simulink model "Linear_Model_Check_mks_4Nov_maininput_cruise"  (R2022b)
settings: Solver=VariableStepAuto  StartTime=0.0  StopTime=3240  FixedStep=0.5  RelTol=1e-6
settings Model: Creator=Mitarbeiter  LastModifiedBy=Mitarbeiter

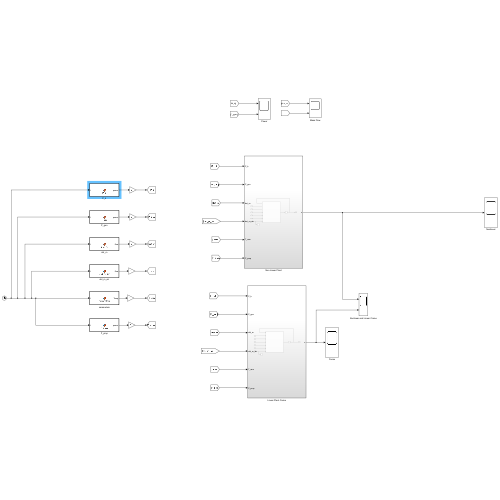
[thumbnail: Simulink's stored preview of the top-level diagram]
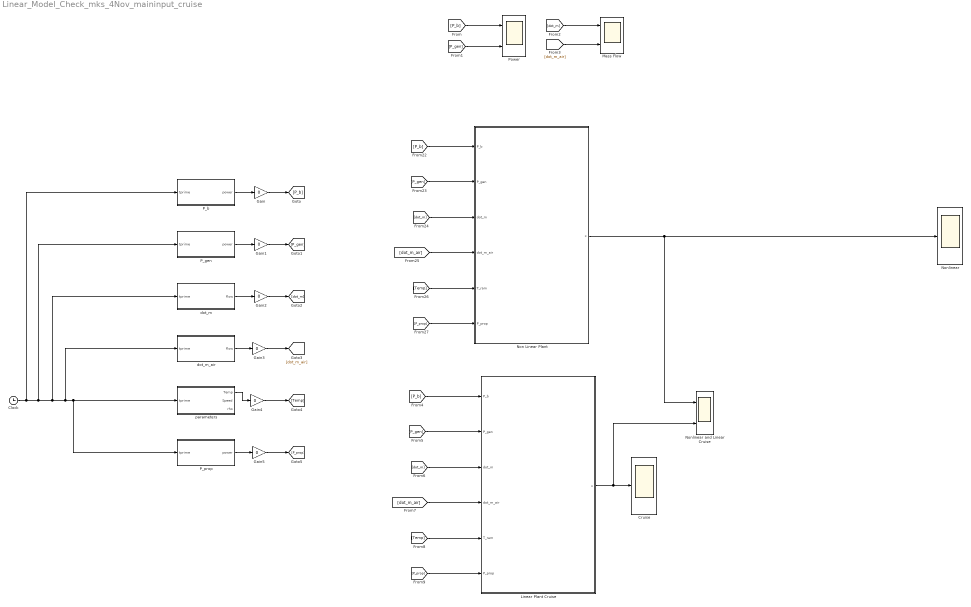
== system Linear_Model_Check_mks_4Nov_maininput_cruise ==
  Clock : Clock
  Cruise : Scope
  Gain{,1..5} (6 alike) : Gain  Gain=0
  Linear Plant Cruise : Subsystem
  Mass Flow : Scope  NumInputPorts=2
  Non Linear Plant : Subsystem
  Nonlinear : Scope
  Nonlinear and Linear Cruise : Scope  NumInputPorts=2
  P_b : MATLAB Function  TreatAsAtomicUnit=on
  P_gen : MATLAB Function  TreatAsAtomicUnit=on
  P_prop : MATLAB Function  TreatAsAtomicUnit=on
  Power : Scope  NumInputPorts=2
  dot_m : MATLAB Function  TreatAsAtomicUnit=on
  dot_m_air : MATLAB Function  TreatAsAtomicUnit=on
  parameters : MATLAB Function  TreatAsAtomicUnit=on
  wires:
  [P_b] -> Power/1
  [P_gen] -> Power/2
  [dot_m] -> Mass Flow/1
  [dot_m_air] -> Mass Flow/2
  [P_b] -> Linear Plant Cruise/1(P_b)
  [dot_m] -> Linear Plant Cruise/3(dot_m)
  Linear Plant Cruise/1(x) -> Nonlinear and Linear Cruise/2, Cruise/1
  [Temp] -> Linear Plant Cruise/5(T_ram)
  [P_prop] -> Linear Plant Cruise/6(P_prop)
  [dot_m_air] -> Linear Plant Cruise/4(dot_m_air)
  [P_gen] -> Linear Plant Cruise/2(P_gen)
  Gain5/1 -> [P_prop]
  P_b/1(power) -> Gain/1
  Gain2/1 -> [dot_m]
  Gain/1 -> [P_b]
  Gain1/1 -> [P_gen]
  P_gen/1(power) -> Gain1/1
  Gain3/1 -> [dot_m_air]
  P_prop/1(power) -> Gain5/1
  parameters/1(Temp) -> Gain4/1
  Clock/1 -> P_b/1(tprime), P_gen/1(tprime), dot_m/1(tprime), dot_m_air/1(tprime), parameters/1(tprime), P_prop/1(tprime)
  Gain4/1 -> [Temp]
  dot_m/1(flow) -> Gain2/1
  dot_m_air/1(flow) -> Gain3/1
  [P_b] -> Non Linear Plant/1(P_b)
  [dot_m] -> Non Linear Plant/3(dot_m)
  Non Linear Plant/1(x) -> Nonlinear and Linear Cruise/1, Nonlinear/1
  [Temp] -> Non Linear Plant/5(T_ram)
  [P_prop] -> Non Linear Plant/6(P_prop)
  [dot_m_air] -> Non Linear Plant/4(dot_m_air)
  [P_gen] -> Non Linear Plant/2(P_gen)

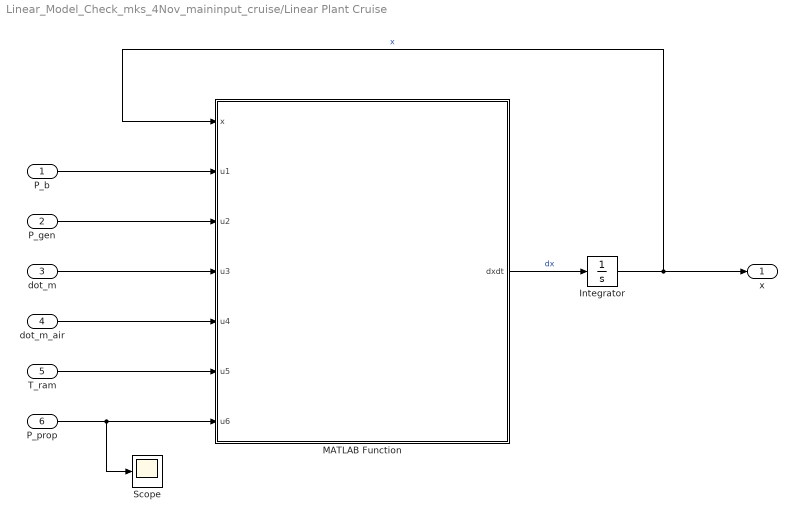
== system Linear_Model_Check_mks_4Nov_maininput_cruise/Linear Plant Cruise ==
  P_b : Inport
  P_gen : Inport  Port=2
  dot_m : Inport  Port=3
  dot_m_air : Inport  Port=4
  T_ram : Inport  Port=5
  P_prop : Inport  Port=6
  Integrator : Integrator  InitialCondition=[52814776030872794621339/2111078349043945281000; 104094200346052350023/4282106184673317000; 0.95; 7429519190417529794477/301582621291992183000; 14970426814841764289/611729454953331000; 62413813461003262061339/2111078349043945281000; 115709353125739950023/4282106184673317000; 1317031521595249/55809639171000; 192210910256741628225757/6125247032447703303000; 18157083865504564289/611729454953331000; 1317031521595249/55809639171000; 29037669531913/1240214203800; 1405698391771/60204573000];
  MATLAB Function : MATLAB Function  TreatAsAtomicUnit=on
  Scope : Scope
  x : Outport
  wires:
  MATLAB Function/1(dxdt) -> Integrator/1  "dx"
  Integrator/1 -> x/1, MATLAB Function/1(x)  "x"
  P_prop/1 -> Scope/1, MATLAB Function/7(u6)
  P_b/1 -> MATLAB Function/2(u1)
  P_gen/1 -> MATLAB Function/3(u2)
  dot_m/1 -> MATLAB Function/4(u3)
  dot_m_air/1 -> MATLAB Function/5(u4)
  T_ram/1 -> MATLAB Function/6(u5)

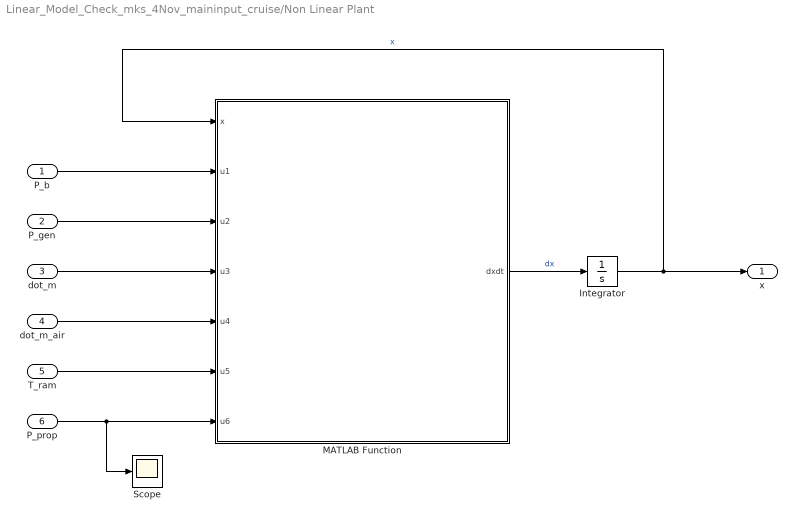
== system Linear_Model_Check_mks_4Nov_maininput_cruise/Non Linear Plant ==
  P_b : Inport
  P_gen : Inport  Port=2
  dot_m : Inport  Port=3
  dot_m_air : Inport  Port=4
  T_ram : Inport  Port=5
  P_prop : Inport  Port=6
  Integrator : Integrator  InitialCondition=[93988057444394599308387229/4422589792359066198000000; 14175896344014406900981/690059259222822000000; 0.95; 642296550198010131218710603/30958128546513463386000000; 99794188918686328306867/4830414814559754000000; 20; 748871653711516104483208603/30958128546513463386000000; 109523475430206270118867/4830414814559754000000; 20; 114489338227757388521/5840888530302000000; 20; 1232797079008717771442215271/48366943538186816802000000; 118698981952749594118867/4830414814559754000000; 114489338227757388521/5840888530302000000; 1053909433374709813/54082301206500000; 8752431102689/450060759000]
  MATLAB Function : MATLAB Function  TreatAsAtomicUnit=on
  Scope : Scope
  x : Outport
  wires:
  MATLAB Function/1(dxdt) -> Integrator/1  "dx"
  Integrator/1 -> x/1, MATLAB Function/1(x)  "x"
  P_prop/1 -> Scope/1, MATLAB Function/7(u6)
  P_b/1 -> MATLAB Function/2(u1)
  P_gen/1 -> MATLAB Function/3(u2)
  dot_m/1 -> MATLAB Function/4(u3)
  dot_m_air/1 -> MATLAB Function/5(u4)
  T_ram/1 -> MATLAB Function/6(u5)

== matlab function Linear_Model_Check_mks_4Nov_maininput_cruise/Linear Plant Cruise/MATLAB Function ==
  data: x input; dxdt output; u1 input; u2 input; u3 input; u4 input; u5 input; u6 input
function dxdt = fcn(x,u1,u2,u3,u4,u5,u6)

u = [u1;u2;u3;u4;u5;u6];
dxdt = aircraft_dynamics_linear_cruise(x,u);

== matlab function Linear_Model_Check_mks_4Nov_maininput_cruise/P_b ==
  data: tprime input; power output
function power = P_b_0to3240(tprime)
% Rebase original profile window: new t' in [0, 3240] corresponds to original t = t' + 421

    % --- Power values (same as your original code) ---
    power_values = [541728.972461324, 525434.547259656, 484698.484257782, ...
                    443962.421182278, 403226.358083855, 362490.295190934, ...
                    321754.232292711, 281018.169380235, 240282.106417171, ...
                    199546.043463649, 158809.980492022, 118073.917524794, ...
                    77337.8545513178, 36601.7915815174, 4012.94120061964, ...
                    4012.94120060897, 4012.94120058611, 4012.94120055903, ...
                    4012.94120053569, 4012.94120052215, 4012.94120051169, ...
                    4012.94120050506, 4012.94120050103, 4012.94120049878, ...
                    4012.94120049977, 4012.94120050145, 4012.94120050538, ...
                    4012.94120051198, 4012.94120052045, 4012.94120053546, ...
                    4012.94120055757, 4012.94120058035, 4012.94120057094, ...
                    9.73312208790910e-10, -3.25790856001986e-10, ...
                    -7.33764827360896e-10, -3.22870604452897e-11, ...
                    -2.89901400312855e-11, -6.19593223381754e-11, ...
                    -4.77143652162351e-10, 3.07295526727322e-10, ...
                    -5.97594860992170e-10, 7.70455739254353e-10, ...
                    -4.62243586863996e-11, 65143.2880368747];

    % --- Corresponding time samples (same as your original code) ---
    time_vector = 1:100:4500;

    % Validate input in the new domain [0, 3240]
    if any(tprime(:) < 0 | tprime(:) > 3240)
        error('t'' must be within 0 to 3240 seconds.');
    end

    % Build spline on original samples and evaluate at shifted time t = t' + 421
    spline_fit = spline(time_vector, power_values);
    power = ppval(spline_fit, tprime + 421);
end

== matlab function Linear_Model_Check_mks_4Nov_maininput_cruise/P_gen ==
  data: tprime input; power output
function power = P_gen_0to3240(tprime)
% New domain: t' in [0, 3240] corresponds to original t = t' + 421

    % --- Your original power samples ---
    power_values = [1560823.08194895, 1546158.09929008, 1509495.64264034, ...
                    1472833.18607241, 1436170.72952995, 1399508.27275915, ...
                    1362845.81599425, 1326183.35924518, 1289520.90255232, ...
                    1252858.44584885, 1216195.98916551, 1179533.53247727, ...
                    1142871.07579598, 1106208.61911061, 1076878.65376792, ...
                    1076878.65376794, 1076878.65376796, 1076878.65376799, ...
                    1076878.65376802, 1076878.65376803, 1076878.65376804, ...
                    1076878.65376805, 1076878.65376806, 1076878.65376806, ...
                    1076878.65376806, 1076878.65376806, 1076878.65376805, ...
                    1076878.65376804, 1076878.65376803, 1076878.65376802, ...
                    1076878.65376799, 1076878.65376797, 1076878.65376798, ...
                    1032182.62799974, 950257.879125699, 868333.130251657, ...
                    786408.381377613, 704483.632503570, 622558.883629528, ...
                    540634.134755485, 458709.385881442, 376784.637007400, ...
                    294859.888133355, 212935.139259313, 58628.9592331873];

    % --- Your original time vector (1,101,...,4401) ---
    time_vector = 1:100:4500;

    % Validate input in the new domain [0, 3240]
    if any(tprime(:) < 0 | tprime(:) > 3240)
        error('t'' must be within 0 to 3240 seconds.');
    end

    % Build spline on the original samples, then evaluate at shifted time t = t' + 421
    spline_fit = spline(time_vector, power_values);
    power = ppval(spline_fit, tprime + 421);
end

== matlab function Linear_Model_Check_mks_4Nov_maininput_cruise/P_prop ==
  data: tprime input; power output
function power = P_prop_0to3240(tprime)
% Map new domain t' ∈ [0, 3240] to original t = t' + 421 and call your original code.
    if any(tprime(:) < 0 | tprime(:) > 3240)
        error('t'' must be within 0 to 3240 seconds.');
    end
    power = P_prop_original(tprime + 421);
end

%% Your original function (unchanged)
function power = P_prop_original(t)
    T_off = 60;
    t_cruise = 420;
    t_descent = 3660;
    t_landing = 4020;
    t_taxi = 4080;
    t_final = 4440;
    
    step = 636e3;
    P_slope_1 = (262e3 - 636e3)/(t_cruise - T_off);
    P_slope_2 = (114e3 - 262e3)/(t_landing - t_descent);
    P_slope_3 = (158e3 - 114e3)/(t_taxi - t_landing);
    P_slope_4 = (40e3 - 158e3)/(t_final - t_taxi);
    
    p_ramp1 = zeros(size(t));
    p_ramp1(t >= T_off) = P_slope_1 * (t(t >= T_off) - T_off);
    
    p_ramp2 = zeros(size(t));
    p_ramp2(t >= t_cruise) = -P_slope_1 * (t(t >= t_cruise) - t_cruise);
    
    p_ramp3 = zeros(size(t));
    p_ramp3(t >= t_descent) = P_slope_2 * (t(t >= t_descent) - t_descent);
    
    p_ramp4 = zeros(size(t));
    p_ramp4(t >= t_landing) = (P_slope_3 - P_slope_2) * (t(t >= t_landing) - t_landing);
    
    p_ramp5 = zeros(size(t));
    p_ramp5(t >= t_taxi) = (P_slope_4 - P_slope_3) * (t(t >= t_taxi) - t_taxi);
    
    power = step + p_ramp1 + p_ramp2 + p_ramp3 + p_ramp4 + p_ramp5;
    power(power < 0) = 0;
end

== matlab function Linear_Model_Check_mks_4Nov_maininput_cruise/dot_m ==
  data: tprime input; flow output
function flow = dot_m_0to3240(tprime)
    % Original samples (kept as-is)
    power_values = [0.904165131160427, 1.62335959482857, 1.97415345554372, ...
                    2.87737856692485, 3.93386755649844, 4.17049006426838, ...
                    3.96224826445125, 3.84633136696794, 3.73843209854831, ...
                    3.62816620139765, 3.51470105395037, 3.39795514134232, ...
                    3.27785630468602, 3.15345777233773, 3.04616198439548, ...
                    3.03635175832522, 2.98312074354866, 2.91947217209040, ...
                    2.86878591164222, 2.83212849923799, 2.80518126603719, ...
                    2.78469068203536, 2.76888505493890, 2.75675815114367, ...
                    2.74763217287481, 2.74096591488524, 2.73636304275517, ...
                    2.73354386559958, 2.73235420493226, 2.73274273164412, ...
                    2.73475441155951, 2.73847704472223, 2.74398498698495, ...
                    2.64313697414983, 2.45549965647436, 2.26040185709996, ...
                    2.23930438794837, 1.99924539905101, 1.61176185199414, ...
                    1.31895743051123, 1.30916014023536, 1.07782805041202, ...
                    0.848496416787671, 0.620762639063214, -5.77778983316171e-34];

    % Original time stamps (kept as-is)
    time_vector = 1:100:4500;

    % New-domain guard
    if any(tprime(:) < 0 | tprime(:) > 3240)
        error('t'' must be within 0 to 3240 seconds.');
    end

    % Interpolate with the original spline, evaluated at shifted time t = t' + 421
    spline_fit = spline(time_vector, power_values);
    flow = ppval(spline_fit, tprime + 421);
end

== matlab function Linear_Model_Check_mks_4Nov_maininput_cruise/dot_m_air ==
  data: tprime input; flow output
function flow = dot_m_air_0to3240(tprime)
    % Original samples (kept as-is)
    power_values = [0.370775472872228, 4.14655917085228, 10.2236066715828, ...
                    15.9335661862365, 19.0351731908349, 16.9149763039733, ...
                    13.1623042033400, 10.7569435504486, 8.94905877526484, ...
                    7.51589529502896, 6.36393337822089, 5.39660249912924, ...
                    4.60743235399543, 4.39417963045294, 4.45647923355531, ...
                    4.36949731785185, 4.31573725145724, 4.26746478317914, ...
                    4.22732179826729, 4.19595415374334, 4.17143491891122, ...
                    4.15169555274063, 4.13523300363972, 4.12099504031059, ...
                    4.10816091872904, 4.09600581489035, 4.08381103149970, ...
                    4.07079463660703, 4.05616667450225, 4.03954164705557, ...
                    4.02160559806096, 4.00355147248531, 3.98237533346872, ...
                    3.81444977989844, 3.58043631849297, 3.43750882096772, ...
                    3.44017594340288, 3.48343898919501, 3.38952732636595, ...
                    3.08055145207970, 2.48510068273254, 1.52973911636135, ...
                    0.577892294612315, 0.0671525631123886, 1.01083847375133e-34];

    % Original time stamps (kept as-is)
    time_vector = 1:100:4500;

    % New-domain guard
    if any(tprime(:) < 0 | tprime(:) > 3240)
        error('t'' must be within 0 to 3240 seconds.');
    end

    % Interpolate with the original spline, evaluated at shifted time t = t' + 421
    spline_fit = spline(time_vector, power_values);
    flow = ppval(spline_fit, tprime + 421);
end

== matlab function Linear_Model_Check_mks_4Nov_maininput_cruise/Non Linear Plant/MATLAB Function ==
  data: x input; dxdt output; u1 input; u2 input; u3 input; u4 input; u5 input; u6 input
function dxdt = fcn(x,u1,u2,u3,u4,u5,u6)

u = [u1;u2;u3;u4;u5;u6];
dxdt = aircraftDynamicsCT(x,u);

== matlab function Linear_Model_Check_mks_4Nov_maininput_cruise/parameters ==
  data: tprime input; Temp output; Speed output; rho output
function [Temp, Speed, rho] = parameters_0to3240(tprime)
% Map new domain t' ∈ [0, 3240] to original t = t' + 421 and call your original code.
    if any(tprime(:) < 0 | tprime(:) > 3240)
        error('t'' must be within 0 to 3240 seconds.');
    end
    [Temp, Speed, rho] = parameters_original(tprime + 421);
end

%% Your original function (unchanged)
function [Temp, Speed, rho] = parameters_original(t)
    %% Calculates aircraft altitude in ft and m
    T_off = 60;
    t_cruise = 420;
    t_landing = 3660;
    t_final = 4440;

    r_slope = (4000-50)/(t_cruise-T_off);
    r_slope2 =(0-4000)/(t_final-t_landing);
    step = 50;

    r_ramp1 = zeros(size(t));
    r_ramp1(t >= T_off) = r_slope * (t(t >= T_off) - T_off);

    r_ramp2 = zeros(size(t));
    r_ramp2(t >= t_cruise) = -r_slope * (t(t >= t_cruise) - t_cruise);

    r_ramp3 = zeros(size(t));
    r_ramp3(t >= t_landing) = r_slope2 * (t(t >= t_landing) - t_landing);

    h = step + r_ramp1 + r_ramp2 + r_ramp3;
    h(h < 0) = 0;
    h = 0.3048 * h;   % meters

    %% Ambient temperature and speed of sound
    Gamma = 1.4; R = 287.053;
    T_amp = -6.5e-3 * h + 15;                 % °C
    a = sqrt(Gamma * R * (T_amp + 273.15));   % m/s

    %% Aircraft speed → knots → m/s → Mach
    s_slope_1 = 77/60;
    s_slope_2 = (125 - 77) / (t_cruise - T_off);
    s_slope_3 = (78 - 125) / (t_final - t_landing);

    S_ramp  = zeros(size(t));
    S_ramp(t <= T_off) = s_slope_1 * t(t <= T_off);

    S_ramp1 = zeros(size(t));
    S_ramp1(t > T_off & t < t_cruise) = s_slope_2 * (t(t > T_off & t < t_cruise) - T_off) + 77;

    S_ramp2 = zeros(size(t));
    S_ramp2(t >= t_cruise & t <= t_landing) = 125;

    S_ramp3 = zeros(size(t));
    S_ramp3(t > t_landing & t <= t_final) = s_slope_3 * (t(t > t_landing & t <= t_final) - t_landing) + 125;

    S_ramp4 = zeros(size(t));
    S_ramp4(t > t_final) = s_slope_3 * (t(t > t_final) - t_final) + 78;

    knot = S_ramp + S_ramp1 + S_ramp2 + S_ramp3 + S_ramp4;  % knots
    knot = 0.5144 * knot;        % m/s
    Mach = knot ./ a;

    Speed = Mach * 343;          % m/s (kept as in your code)
    %% Ram temperature
    Temp = T_amp .* (1 + Mach.^2 * ((Gamma - 1)/2));

    %% Pressure altitude and density
    P0 = 101325;                                     % Pa
    P  = P0 * (1 - 2.25577e-5 * h).^5.25588;         % Pa
    rho = P ./ (R * (T_amp + 273.15));               % kg/m^3
end
